simulink model "mpc_rf_boiler_open_loop"  (R2017a)
settings: Solver=FixedStepAuto  StartTime=0.0  StopTime=simTime  FixedStep=Dt  RelTol=1e-3  EnableMultiTasking=on
values from neighbouring files (symbols this model uses):
  beta = 100    [mpcGASimulink_2205_dummy.m]    (also in mpc_design_parameters_0206.mat = [0 0 0]; mpc_design_parameters_0606.mat = [0 0 0]; mpc_design_parameters_0706.mat = [0.0001 0.0001 0.0001]; mpc_design_parameters_2805.mat = 1)
  bFilter = fir1(10,0.8,kaiser(11,6))    [mpcBoiler_0206.m]    (also in mpcBoiler_closed_loop_0206.m = 1; mpcBoiler_open_loop_0206.m = 1)
  controlClosedLoop = 1    [mpcBoiler_open_loop_0206.m]
  D0 = 35.783396242    [cic2017_fase1_boiler.mat]    (also in compare_rf_boiler.m = 35.7834; control_Caldera_3004.m = 35.7834; mpcGASimulink_2205_dummy.m = 35.7834; mpc_design_parameters_0206.mat = 35.7834)
  Dt = 1    [compare_rf_boiler.m]    (also in control_Caldera_3004.m = 0.5; mpcBoiler_0206.m; mpcBoiler_2805.m; mpcBoiler_closed_loop_0206.m)
  GAParameters = [100 100 75 1e-06 3 5 9]    [mpc_design_parameters_0206.mat]    (also in mpc_design_parameters_0606.mat = [200 100 75 1e-06 3 10 9]; mpc_design_parameters_0706.mat = [200 50 37 1e-06 3 10 9]; mpc_design_parameters_2805.mat = [100 100 50 1e-06 3 3])
  lambdaMatrix = 100*ones(numOutputs,N_y)    [mpcGASimulink_2205_dummy.m]    (also in mpc_design_parameters_0206.mat = [0 0 0 0 0 0 0 0 0 0 0 0 ... (30 elements, 3x10)]; mpc_design_parameters_0606.mat = [0 0 0 0 0 0 0 0 0 0 0 0 ... (30 elements, 3x10)]; mpc_design_parameters_0706.mat = [0.0001 0.0001 0.0001 0.0001 0.0001 0.0001 0.0001 0.0001 0.0; mpc_design_parameters_2805.mat = [1 1 1 1 1 1 1 1 1 1 1 1 ... (15 elements, 3x5)])
  lBounds = [0 0 0 -2*ones(1,numOutputs*N_u)]    [mpcGASimulink_2205_dummy.m]    (also in mpc_design_parameters_0206.mat = [-5 -5 -5 -5 -5 -5 -5 -5 -5]; mpc_design_parameters_0606.mat = [-5 -5 -5 -5 -5 -5 -5 -5 -5]; mpc_design_parameters_0706.mat = [-5 -5 -5 -5 -5 -5 -5 -5 -5]; mpc_design_parameters_2805.mat = [-15 -15 -15])
  maxDDelay = maxDelay(3)    [compare_rf_boiler.m]    (also in mpcGASimulink_2205_dummy.m = max(max(nc)); mpc_design_parameters_0206.mat = 2; mpc_design_parameters_0606.mat = 2; mpc_design_parameters_0706.mat = 2)
  maxUDelay = maxDelay(2)    [compare_rf_boiler.m]    (also in mpcGASimulink_2205_dummy.m = max(max(nb)); mpc_design_parameters_0206.mat = 2; mpc_design_parameters_0606.mat = 2; mpc_design_parameters_0706.mat = 2)
  maxYDelay = maxDelay(1)    [compare_rf_boiler.m]    (also in mpcGASimulink_2205_dummy.m = max(na); mpc_design_parameters_0206.mat = 4; mpc_design_parameters_0606.mat = 4; mpc_design_parameters_0706.mat = 4)
  na = [delayYMatrix(2,2);delayYMatrix(2,2);delayYMatrix(3,3)]    [mpcGASimulink_2205_dummy.m]    (also in mpc_design_parameters_0206.mat = [4 4 4]; mpc_design_parameters_0606.mat = [4 4 4]; mpc_design_parameters_0706.mat = [4 4 4]; mpc_design_parameters_2805.mat = [4 3 4])
  nb = delayUMatrix(:,2:end)    [mpcGASimulink_2205_dummy.m]    (also in mpc_design_parameters_0206.mat = [1  1  1; 2  2  2; 2  2  2]; mpc_design_parameters_0606.mat = [1  1  1; 2  2  2; 2  2  2]; mpc_design_parameters_0706.mat = [1  1  1; 2  2  2; 2  2  2]; mpc_design_parameters_2805.mat = [1  1  1; 1  1  1; 1  2  1])
  nc = delayUMatrix(:,1)    [mpcGASimulink_2205_dummy.m]    (also in mpc_design_parameters_0206.mat = [1 2 2]; mpc_design_parameters_0606.mat = [1 2 2]; mpc_design_parameters_0706.mat = [1 2 2]; mpc_design_parameters_2805.mat = [1 1 2])
  nPredictors = [8 12 12]    [compare_rf_boiler.m]    (also in mpcGASimulink_2205_dummy.m = 10*ones(1,3); mpc_design_parameters_0206.mat; mpc_design_parameters_0606.mat; mpc_design_parameters_0706.mat)
  nTrees = ones(1,numCV)*100    [compare_rf_boiler.m]    (also in mpcGASimulink_2205_dummy.m = ones(1,3)*100; mpc_design_parameters_0206.mat = [100 100 100]; mpc_design_parameters_0606.mat = [100 100 100]; mpc_design_parameters_0706.mat = [100 100 100])
  qMatrix = ones(numOutputs,N_y-1)    [mpcGASimulink_2205_dummy.m]    (also in mpc_design_parameters_0206.mat = [0 1 1 0 1 1 0 1 1 0 1 1 ... (27 elements, 3x9)]; mpc_design_parameters_0606.mat = [0 1 1 0 1 1 0 1 1 0 1 1 ... (27 elements, 3x9)]; mpc_design_parameters_0706.mat = [1e-05 1 1 1e-05 1 1 1e-05 1 1 1e-05 1 1 ... (27 elements, 3; mpc_design_parameters_2805.mat = [1000  1000  1000  1000; 1000  1000  1000  1000; 1000  1000 )
  rMatrix = ones(numMV,N_u)    [mpcGASimulink_2205_dummy.m]    (also in mpc_design_parameters_0206.mat = [1  1  1; 1  1  1; 100  100  100]; mpc_design_parameters_0606.mat = [1  1  1; 1  1  1; 0.01  0.01  0.01]; mpc_design_parameters_0706.mat = [1  1  1; 1  1  1; 0.01  0.01  0.01]; mpc_design_parameters_2805.mat = [1 1 1])
  tau_C = 12    [mpcBoiler_0206.m]    (also in mpcBoiler_2805.m; mpcBoiler_closed_loop_0206.m; mpcBoiler_open_loop_0206.m; mpcGASimulink_2205_dummy.m = 60)
  tau_R = 5    [compare_rf_boiler.m]    (also in delayParameters_0706.mat; delayParameters_2805.mat; mpcBoiler_0206.m; mpcBoiler_2805.m)
  U0 = [32.9815865199 46.2282063472 25.3416381967]    [cic2017_fase1_boiler.mat]    (also in compare_rf_boiler.m = [32.9816   46.2282   25.3416]; control_Caldera_3004.m = [32.9816   46.2282   25.3416]; mpcGASimulink_2205_dummy.m = [32.9816   46.2282   25.3416]; mpc_design_parameters_0206.mat = [32.9816 46.2282 25.3416])
  uBounds = [1 1 2 2*ones(1,numOutputs*N_u)]    [mpcGASimulink_2205_dummy.m]    (also in mpc_design_parameters_0206.mat = [5 5 5 5 5 5 5 5 5]; mpc_design_parameters_0606.mat = [5 5 5 5 5 5 5 5 5]; mpc_design_parameters_0706.mat = [5 5 5 5 5 5 5 5 5]; mpc_design_parameters_2805.mat = [15 15 15])
  uLims = [0 0 0 0 0 0 0 0 0 100 100 100 ... (18 elements, 3x3x2)]    [mpc_design_parameters_0206.mat]    (also in mpc_design_parameters_0606.mat; mpc_design_parameters_0706.mat; mpc_design_parameters_2805.mat = [0 0 0 100 100 100])
  Y0 = [41.4119839556 28.7552838432 38.6036799989]    [cic2017_fase1_boiler.mat]    (also in compare_rf_boiler.m = [41.4120   28.7553   38.6037]; control_Caldera_3004.m = [41.4120   28.7553   38.6037]; mpcGASimulink_2205_dummy.m = [41.4120   28.7553   38.6037]; mpc_design_parameters_0206.mat = [41.412 28.7553 38.6037])
  yLims = cat(3,yLowLims,yHighLims)    [mpcGASimulink_2205_dummy.m]    (also in mpc_design_parameters_0206.mat = [0 27.317535 0 0 27.317535 0 0 27.317535 0 0 27.317535 0 ...; mpc_design_parameters_0606.mat = [0 27.317535 0 0 27.317535 0 0 27.317535 0 0 27.317535 0 ...; mpc_design_parameters_0706.mat = [0 27.317535 0 0 27.317535 0 0 27.317535 0 0 27.317535 0 ...; mpc_design_parameters_2805.mat = [0 27.317535 0 0 27.317535 0 0 27.317535 0 0 27.317535 0 ...)
settings Model: Creator=Pablo Diaz  LastModifiedBy=Felipe
settings OptimizationCC: LifeSpan=inf
settings DebuggingCC: SFUnexpectedBacktrackingDiag=warning  SFNoUnconditionalDefaultTransitionDiag=warning  SFExecutionAtInitializationDiag=none
settings GRTTargetCC: TargetLangStandard=C89/C90 (ANSI)
settings ConfigComp: CovMetricSettings=dw  CovHtmlReporting=on  CovSaveCumulativeToWorkspaceVar=on  CovSaveSingleToWorkspaceVar=on  CovExternalEMLEnable=off

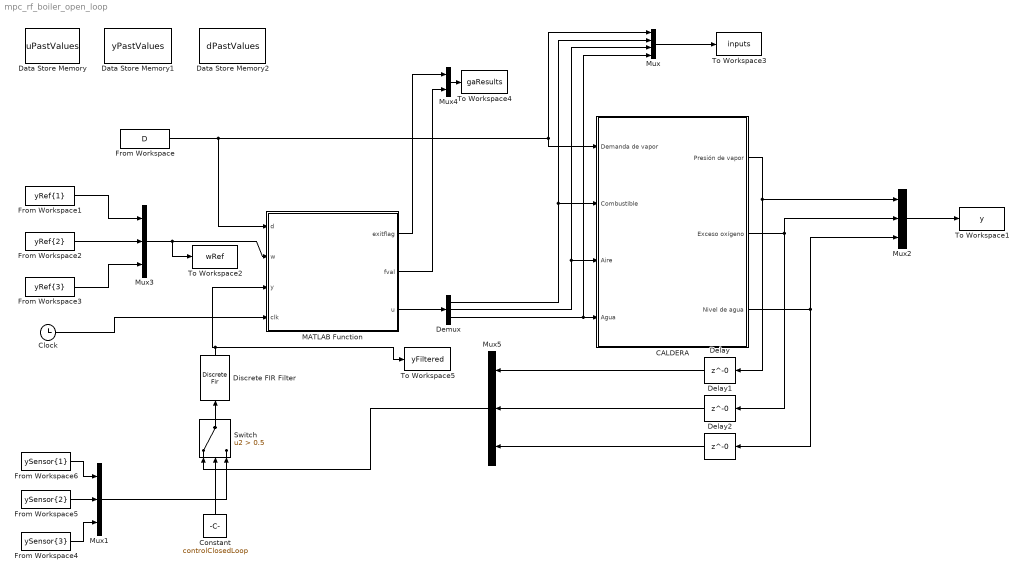
== system mpc_rf_boiler_open_loop ==
  CALDERA : Subsystem
  Clock : Clock
  Constant : Constant  Value=controlClosedLoop
  Data Store Memory : DataStoreMemory  DataStoreName=uPastValues  ReadBeforeWriteMsg=warning  WriteAfterWriteMsg=warning  WriteAfterReadMsg=warning  InitialValue=[U0]'*ones(1,maxUDelay);  VectorParams1D=off  ShowAdditionalParam=off  OutDataTypeStr=double
  Data Store Memory1 : DataStoreMemory  DataStoreName=yPastValues  ReadBeforeWriteMsg=warning  WriteAfterWriteMsg=warning  WriteAfterReadMsg=warning  InitialValue=Y0'*ones(1,maxYDelay)  VectorParams1D=off  ShowAdditionalParam=off  OutDataTypeStr=double
  Data Store Memory2 : DataStoreMemory  DataStoreName=dPastValues  ReadBeforeWriteMsg=warning  WriteAfterWriteMsg=warning  WriteAfterReadMsg=warning  InitialValue=D0'*ones(1,maxDDelay)  VectorParams1D=off  ShowAdditionalParam=off  OutDataTypeStr=double
  Delay : Delay  DelayLength=0  InitialCondition=Y0(1)
  Delay1 : Delay  DelayLength=0  InitialCondition=Y0(2)
  Delay2 : Delay  DelayLength=0  InitialCondition=Y0(3)
  Demux : Demux  Outputs=3
  Discrete FIR Filter : DiscreteFir  Coefficients=bFilter
  From Workspace : FromWorkspace  VariableName=D  SampleTime=Dt  Interpolate=off  OutputAfterFinalValue=Holding final value
  From Workspace1 : FromWorkspace  VariableName=yRef{1}  SampleTime=Dt  Interpolate=off  OutputAfterFinalValue=Holding final value
  From Workspace2 : FromWorkspace  VariableName=yRef{2}  SampleTime=0  Interpolate=off  OutputAfterFinalValue=Holding final value
  From Workspace3 : FromWorkspace  VariableName=yRef{3}  SampleTime=Dt  Interpolate=off  OutputAfterFinalValue=Holding final value
  From Workspace4 : FromWorkspace  VariableName=ySensor{3}  SampleTime=Dt  Interpolate=off  OutputAfterFinalValue=Holding final value
  From Workspace5 : FromWorkspace  VariableName=ySensor{2}  SampleTime=Dt  Interpolate=off  OutputAfterFinalValue=Holding final value
  From Workspace6 : FromWorkspace  VariableName=ySensor{1}  SampleTime=Dt  Interpolate=off  OutputAfterFinalValue=Holding final value
  MATLAB Function : MATLAB Function  TreatAsAtomicUnit=on
  Mux : Mux
  Mux{1..3,5} (4 alike) : Mux  Inputs=3
  Mux4 : Mux  Inputs=2
  Switch : Switch  Criteria=u2 > Threshold  Threshold=0.5
  To Workspace1 : ToWorkspace  VariableName=y  SaveFormat=Structure With Time  SampleTime=-1
  To Workspace2 : ToWorkspace  VariableName=wRef  SaveFormat=Structure With Time  SampleTime=-1
  To Workspace3 : ToWorkspace  VariableName=inputs  SaveFormat=Structure With Time  SampleTime=-1
  To Workspace4 : ToWorkspace  VariableName=gaResults  SaveFormat=Structure With Time  SampleTime=-1
  To Workspace5 : ToWorkspace  VariableName=yFiltered  SaveFormat=Structure With Time  SampleTime=-1
  wires:
  Mux/1 -> To Workspace3/1
  MATLAB Function/3(u) -> Demux/1
  Mux3/1 -> To Workspace2/1, MATLAB Function/2(w)
  From Workspace1/1 -> Mux3/1
  From Workspace2/1 -> Mux3/2
  From Workspace3/1 -> Mux3/3
  MATLAB Function/1(exitflag) -> Mux4/1
  Mux4/1 -> To Workspace4/1
  MATLAB Function/2(fval) -> Mux4/2
  Clock/1 -> MATLAB Function/4(clk)
  Discrete FIR Filter/1 -> MATLAB Function/3(y), To Workspace5/1
  From Workspace5/1 -> Mux1/2
  From Workspace6/1 -> Mux1/1
  From Workspace4/1 -> Mux1/3
  Delay/1 -> Mux5/1
  Delay1/1 -> Mux5/2
  Delay2/1 -> Mux5/3
  Demux/3 -> Mux/4, CALDERA/4(Agua)
  CALDERA/2(Exceso oxígeno) -> Mux2/2, Delay1/1
  Mux2/1 -> To Workspace1/1
  CALDERA/3(Nivel de agua) -> Mux2/3, Delay2/1
  Demux/2 -> Mux/3, CALDERA/3(Aire)
  From Workspace/1 -> MATLAB Function/1(d), Mux/1, CALDERA/1(Demanda de vapor)
  Demux/1 -> Mux/2, CALDERA/2(Combustible)
  CALDERA/1(Presión de vapor) -> Delay/1, Mux2/1
  Switch/1 -> Discrete FIR Filter/1
  Constant/1 -> Switch/2
  Mux5/1 -> Switch/1
  Mux1/1 -> Switch/3

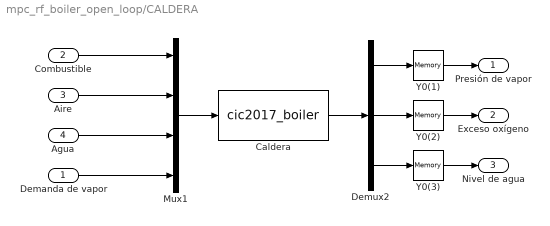
== system mpc_rf_boiler_open_loop/CALDERA ==
  Demanda de vapor : Inport
  Combustible : Inport  Port=2
  Aire : Inport  Port=3
  Agua : Inport  Port=4
  Caldera : S-Function  FunctionName=cic2017_boiler  Parameters=Y0,[U0 D0]  SFunctionDeploymentMode=off  EnableBusSupport=off
  Demux2 : Demux  Outputs=3
  Mux1 : Mux
  Y0(1) : Memory  X0=Y0(1)
  Y0(2) : Memory  X0=Y0(2)
  Y0(3) : Memory  X0=Y0(3)
  Presión de vapor : Outport
  Exceso oxígeno : Outport  Port=2
  Nivel de agua : Outport  Port=3
  wires:
  Caldera/1 -> Demux2/1
  Aire/1 -> Mux1/2
  Agua/1 -> Mux1/3
  Demanda de vapor/1 -> Mux1/4
  Combustible/1 -> Mux1/1
  Mux1/1 -> Caldera/1
  Demux2/1 -> Y0(1)/1
  Demux2/2 -> Y0(2)/1
  Demux2/3 -> Y0(3)/1
  Y0(1)/1 -> Presión de vapor/1
  Y0(2)/1 -> Exceso oxígeno/1
  Y0(3)/1 -> Nivel de agua/1

== matlab function mpc_rf_boiler_open_loop/MATLAB Function ==
  data: exitflag output; fval output; d input; w input; y input; clk input; u output; qMatrix parameter; rMatrix parameter; lambdaMatrix parameter; beta parameter; yLims parameter; lBounds parameter; uBounds parameter; nTrees parameter; nPredictors parameter; na parameter; nb parameter; nc parameter; yPastValues data_store_memory; uPastValues data_store_memory; dPastValues data_store_memory; tau_R parameter; tau_C parameter; uLims parameter; GAParameters parameter
function [exitflag, fval, u] = MPC_RF(d, w, y, clk,...
                                    qMatrix, rMatrix, lambdaMatrix, beta,...
                                    yLims, lBounds, uBounds, ...
                                    nTrees, nPredictors, na, nb, nc,...
                                    tau_R, tau_C,...
                                    uLims,GAParameters)
coder.extrinsic('mpc_wrapper_ga');
global yPastValues
global uPastValues
global dPastValues
[m,N_u] = size(rMatrix);
nPopulation = GAParameters(1);
%% Extrinsic pre declaration
UNow = [0 0 0]';
fval = NaN;
exitflag = NaN;
population = zeros(nPopulation,m*N_u); % Change after
scores = zeros(nPopulation,1);
%%
if rem(clk,tau_R) == 0
    % Sample time for tau_R has been hit
    
    % Refresh past sequences of Y and D with new measured value
    yPastValues(:,2:end) = yPastValues(:,1:(end-1));
    dPastValues(:,2:end) = dPastValues(:,1:(end-1));
    yPastValues(:,1) = y;
    dPastValues(:,1) = d;
    if rem(clk,tau_C*tau_R) == 0
        % Compute optimal MV values (saturated inside)
        wMatrix = mpc_generate_w_matrix(w,qMatrix);
        [UNow,fval,exitflag,population,scores] = mpc_wrapper_ga(yPastValues,uPastValues,dPastValues,...
                                                              qMatrix,rMatrix,lambdaMatrix,beta,wMatrix,...
                                                              yLims,uLims,lBounds,uBounds,...
                                                              nTrees,nPredictors,na,nb,nc,...
                                                              GAParameters);
    else
        % Keep MV in past values if no MPC computation was required
        UNow = uPastValues(:,1);
    end
    uPastValues(:,2:end) = uPastValues(:,1:(end-1));
    uPastValues(:,1) = UNow;
else
    % Keep MV in past values if not
    UNow = uPastValues(:,1);
end
u = UNow;
